simulink model "npc_controller"  (R2022a)
settings: Solver=FixedStepDiscrete  StartTime=0.0  StopTime=20  RelTol=1e-3  EnableMultiTasking=on
undefined symbols (not defined in the file): CAN_O_INT, CANA_BASE, Down, GPTRIP1SEL, GPTRIP2SEL, GPTRIP3SEL, Tsw, TZ1, TZ2, TZ3, Up
libraries: simulink x147, hdlsllib x90, c2802xlib x34, c2837xDlib x20, c280xlib x12, canmsglib x9, c2838xlib x8, idelinklib_common x3, c2806xlib x2, slpidlib x2, c28004xlib x2, c281xlib x2
(part 16 of 42)

== system npc_controller/IDLE_AND_TIMER/codegen/INITIALIZATION/clb ==
  note: // Enabling EPWM1 to enable CLB1
      | SysCtl_enablePeripheral(SYSCTL_PERIPH_CLK_EPWM1);
      | CLB_enableCLB(CLB1_BASE);
      | initTILE0(CLB1_BASE);
      |
      | // Select Global input instead of local input for all CLB IN
      | CLB_configLocalInputMux(CLB1_BASE, CLB_IN0, CLB_LOCAL_IN_MUX_GLOBAL_IN);
      | CLB_configLocalInputMux(CLB1_BASE, CLB_IN1, CLB_LOCAL_IN_MUX_GLOBAL_IN);
      | CLB_configLocalInputMux(CLB1_BASE, CLB_IN2, CLB_LOCAL_IN_MUX_GLOBAL_IN);
      | CLB_configLocalInputMux(CLB1_BASE, CLB_IN3, CLB_LOCAL_IN_MUX_GLOBAL_IN);
      | CLB_configLocalInputMux(CLB1_BASE, CLB_IN4, CLB_LOCAL_IN_MUX_GLOBAL_IN);
      | CLB_configLocalInputMux(CLB1_BASE, CLB_IN5, CLB_LOCAL_IN_MUX_GLOBAL_IN);
      | CLB_configLocalInputMux(CLB1_BASE, CLB_IN6, CLB_LOCAL_IN_MUX_GLOBAL_IN);
      | CLB_configLocalInputMux(CLB1_BASE, CLB_IN7, CLB_LOCAL_IN_MUX_GLOBAL_IN);
      |
      | // Select AUXSIG for CLBx, IN0/1/2
      | CLB_configGlobalInputMux(CLB1_BASE, CLB_IN0, CLB_GLOBAL_IN_MUX_CLB_AUXSIG0);
      | CLB_configGlobalInputMux(CLB1_BASE, CLB_IN1, CLB_GLOBAL_IN_MUX_CLB_AUXSIG1);
      | CLB_configGlobalInputMux(CLB1_BASE, CLB_IN2, CLB_GLOBAL_IN_MUX_EPWM1B);
      |
      | // Unused inputs below
      | CLB_configGlobalInputMux(CLB1_BASE, CLB_IN3, CLB_GLOBAL_IN_MUX_EPWM1A);
      | CLB_configGlobalInputMux(CLB1_BASE, CLB_IN4, CLB_GLOBAL_IN_MUX_EPWM1A);
      | CLB_configGlobalInputMux(CLB1_BASE, CLB_IN5, CLB_GLOBAL_IN_MUX_EPWM1A);
      | CLB_configGlobalInputMux(CLB1_BASE, CLB_IN6, CLB_GLOBAL_IN_MUX_EPWM1A);
      | CLB_configGlobalInputMux(CLB1_BASE, CLB_IN7, CLB_GLOBAL_IN_MUX_EPWM1A);
      |
      | // Set CLB_IN to mux external
      | CLB_configGPInputMux(CLB1_BASE, CLB_IN0, CLB_GP_IN_MUX_EXTERNAL);
      | CLB_configGPInputMux(CLB1_BASE, CLB_IN1, CLB_GP_IN_MUX_EXTERNAL);
      | CLB_configGPInputMux(CLB1_BASE, CLB_IN2, CLB_GP_IN_MUX_EXTERNAL);
      |
      | // Set unused inputs to GP register
      | CLB_configGPInputMux(CLB1_BASE, CLB_IN3, CLB_GP_IN_MUX_GP_REG);
      | CLB_configGPInputMux(CLB1_BASE, CLB_IN4, CLB_GP_IN_MUX_GP_REG);
      | CLB_configGPInputMux(CLB1_BASE, CLB_IN5, CLB_GP_IN_MUX_GP_REG);
      | CLB_configGPInputMux(CLB1_BASE, CLB_IN6, CLB_GP_IN_MUX_GP_REG);
      | CLB_configGPInputMux(CLB1_BASE, CLB_IN7, CLB_GP_IN_MUX_GP_REG);
      |
      | // Configure CLB-XBAR AUXSIG
      | XBAR_setCLBMuxConfig(XBAR_AUXSIG0, XBAR_EPWM_MUX02_CMPSS2_CTRIPH);
      | XBAR_enableCLBMux(XBAR_AUXSIG0, XBAR_MUX02);
      | XBAR_setCLBMuxConfig(XBAR_AUXSIG1, XBAR_EPWM_MUX03_CMPSS2_CTRIPL);
      | XBAR_enableCLBMux(XBAR_AUXSIG1, XBAR_MUX03);
      |
      | // Configure ePWM XBAR
      | XBAR_setEPWMMuxConfig(XBAR_TRIP4, XBAR_EPWM_MUX01_CLB1_OUT4);
      | XBAR_enableEPWMMux(XBAR_TRIP4, XBAR_MUX01);
      | XBAR_setEPWMMuxConfig(XBAR_TRIP5, XBAR_EPWM_MUX03_CLB1_OUT5);
      | XBAR_enableEPWMMux(XBAR_TRIP5, XBAR_MUX03);
  note: // Enabling EPWM1 to enable CLB1
      | SysCtl_enablePeripheral(SYSCTL_PERIPH_CLK_EPWM1);
      | CLB_enableCLB(CLB1_BASE);
      | initTILE0(CLB1_BASE);
      | CLB_enableCLB(CLB2_BASE);
      | initTILE1(CLB2_BASE);
      | CLB_enableCLB(CLB3_BASE);
      | initTILE2(CLB3_BASE);
      |
      | // Select Global input instead of local input for all CLB IN
      | CLB_configLocalInputMux(CLB1_BASE, CLB_IN0, CLB_LOCAL_IN_MUX_GLOBAL_IN);
      | CLB_configLocalInputMux(CLB1_BASE, CLB_IN1, CLB_LOCAL_IN_MUX_GLOBAL_IN);
      | CLB_configLocalInputMux(CLB1_BASE, CLB_IN2, CLB_LOCAL_IN_MUX_GLOBAL_IN);
      | CLB_configLocalInputMux(CLB1_BASE, CLB_IN3, CLB_LOCAL_IN_MUX_GLOBAL_IN);
      | CLB_configLocalInputMux(CLB1_BASE, CLB_IN4, CLB_LOCAL_IN_MUX_GLOBAL_IN);
      | CLB_configLocalInputMux(CLB1_BASE, CLB_IN5, CLB_LOCAL_IN_MUX_GLOBAL_IN);
      | CLB_configLocalInputMux(CLB1_BASE, CLB_IN6, CLB_LOCAL_IN_MUX_GLOBAL_IN);
      | CLB_configLocalInputMux(CLB1_BASE, CLB_IN7, CLB_LOCAL_IN_MUX_GLOBAL_IN);
      | CLB_configLocalInputMux(CLB2_BASE, CLB_IN0, CLB_LOCAL_IN_MUX_GLOBAL_IN);
      | CLB_configLocalInputMux(CLB2_BASE, CLB_IN1, CLB_LOCAL_IN_MUX_GLOBAL_IN);
      | CLB_configLocalInputMux(CLB2_BASE, CLB_IN2, CLB_LOCAL_IN_MUX_GLOBAL_IN);
      | CLB_configLocalInputMux(CLB2_BASE, CLB_IN3, CLB_LOCAL_IN_MUX_GLOBAL_IN);
      | CLB_configLocalInputMux(CLB2_BASE, CLB_IN4, CLB_LOCAL_IN_MUX_GLOBAL_IN);
      | CLB_configLocalInputMux(CLB2_BASE, CLB_IN5, CLB_LOCAL_IN_MUX_GLOBAL_IN);
      | CLB_configLocalInputMux(CLB2_BASE, CLB_IN6, CLB_LOCAL_IN_MUX_GLOBAL_IN);
      | CLB_configLocalInputMux(CLB2_BASE, CLB_IN7, CLB_LOCAL_IN_MUX_GLOBAL_IN);
      | CLB_configLocalInputMux(CLB3_BASE, CLB_IN0, CLB_LOCAL_IN_MUX_GLOBAL_IN);
      | CLB_configLocalInputMux(CLB3_BASE, CLB_IN1, CLB_LOCAL_IN_MUX_GLOBAL_IN);
      | CLB_configLocalInputMux(CLB3_BASE, CLB_IN2, CLB_LOCAL_IN_MUX_GLOBAL_IN);
      | CLB_configLocalInputMux(CLB3_BASE, CLB_IN3, CLB_LOCAL_IN_MUX_GLOBAL_IN);
      | CLB_configLocalInputMux(CLB3_BASE, CLB_IN4, CLB_LOCAL_IN_MUX_GLOBAL_IN);
      | CLB_configLocalInputMux(CLB3_BASE, CLB_IN5, CLB_LOCAL_IN_MUX_GLOBAL_IN);
      | CLB_configLocalInputMux(CLB3_BASE, CLB_IN6, CLB_LOCAL_IN_MUX_GLOBAL_IN);
      | CLB_configLocalInputMux(CLB3_BASE, CLB_IN7, CLB_LOCAL_IN_MUX_GLOBAL_IN);
      |
      | // Select AUXSIG for CLBx, IN0/1/2
      | CLB_configGlobalInputMux(CLB1_BASE, CLB_IN0, CLB_GLOBAL_IN_MUX_CLB_AUXSIG0);
      | CLB_configGlobalInputMux(CLB1_BASE, CLB_IN1, CLB_GLOBAL_IN_MUX_CLB_AUXSIG1);
      | CLB_configGlobalInputMux(CLB1_BASE, CLB_IN2, CLB_GLOBAL_IN_MUX_EPWM1B);
      | CLB_configGlobalInputMux(CLB2_BASE, CLB_IN0, CLB_GLOBAL_IN_MUX_CLB_AUXSIG2);
      | CLB_configGlobalInputMux(CLB2_BASE, CLB_IN1, CLB_GLOBAL_IN_MUX_CLB_AUXSIG3);
      | CLB_configGlobalInputMux(CLB2_BASE, CLB_IN2, CLB_GLOBAL_IN_MUX_EPWM3B);
      | CLB_configGlobalInputMux(CLB3_BASE, CLB_IN0, CLB_GLOBAL_IN_MUX_CLB_AUXSIG4);
      | CLB_configGlobalInputMux(CLB3_BASE, CLB_IN1, CLB_GLOBAL_IN_MUX_CLB_AUXSIG5);
      | CLB_configGlobalInputMux(CLB3_BASE, CLB_IN2, CLB_GLOBAL_IN_MUX_EPWM4B);
      |
      | // Unused inputs below
      | CLB_configGlobalInputMux(CLB1_BASE, CLB_IN3, CLB_GLOBAL_IN_MUX_EPWM1A);
      | CLB_configGlobalInputMux(CLB1_BASE, CLB_IN4, CLB_GLOBAL_IN_MUX_EPWM1A);
      | CLB_configGlobalInputMux(CLB1_BASE, CLB_IN5, CLB_GLOBAL_IN_MUX_EPWM1A);
      | CLB_configGlobalInputMux(CLB1_BASE, CLB_IN6, CLB_GLOBAL_IN_MUX_EPWM1A);
      | CLB_configGlobalInputMux(CLB1_BASE, CLB_IN7, CLB_GLOBAL_IN_MUX_EPWM1A);
      | CLB_configGlobalInputMux(CLB2_BASE, CLB_IN3, CLB_GLOBAL_IN_MUX_EPWM1A);
      | CLB_configGlobalInputMux(CLB2_BASE, CLB_IN4, CLB_GLOBAL_IN_MUX_EPWM1A);
      | CLB_configGlobalInputMux(CLB2_BASE, CLB_IN5, CLB_GLOBAL_IN_MUX_EPWM1A);
      | CLB_configGlobalInputMux(CLB2_BASE, CLB_IN6, CLB_GLOBAL_IN_MUX_EPWM1A);
      | CLB_configGlobalInputMux(CLB2_BASE, CLB_IN7, CLB_GLOBAL_IN_MUX_EPWM1A);
      | CLB_configGlobalInputMux(CLB3_BASE, CLB_IN3, CLB_GLOBAL_IN_MUX_EPWM1A);
      | CLB_configGlobalInputMux(CLB3_BASE, CLB_IN4, CLB_GLOBAL_IN_MUX_EPWM1A);
      | CLB_configGlobalInputMux(CLB3_BASE, CLB_IN5, CLB_GLOBAL_IN_MUX_EPWM1A);
      | CLB_configGlobalInputMux(CLB3_BASE, CLB_IN6, CLB_GLOBAL_IN_MUX_EPWM1A);
      | CLB_configGlobalInputMux(CLB3_BASE, CLB_IN7, CLB_GLOBAL_IN_MUX_EPWM1A);
      |
      | // Set CLB_IN to mux external
      | CLB_configGPInputMux(CLB1_BASE, CLB_IN0, CLB_GP_IN_MUX_EXTERNAL);
      | CLB_configGPInputMux(CLB1_BASE, CLB_IN1, CLB_GP_IN_MUX_EXTERNAL);
      | CLB_configGPInputMux(CLB1_BASE, CLB_IN2, CLB_GP_IN_MUX_EXTERNAL);
      | CLB_configGPInputMux(CLB2_BASE, CLB_IN0, CLB_GP_IN_MUX_EXTERNAL);
      | CLB_configGPInputMux(CLB2_BASE, CLB_IN1, CLB_GP_IN_MUX_EXTERNAL);
      | CLB_configGPInputMux(CLB2_BASE, CLB_IN2, CLB_GP_IN_MUX_EXTERNAL);
      | CLB_configGPInputMux(CLB3_BASE, CLB_IN0, CLB_GP_IN_MUX_EXTERNAL);
      | CLB_configGPInputMux(CLB3_BASE, CLB_IN1, CLB_GP_IN_MUX_EXTERNAL);
      | CLB_configGPInputMux(CLB3_BASE, CLB_IN2, CLB_GP_IN_MUX_EXTERNAL);
      |
      | // Set unused inputs to GP register
      | CLB_configGPInputMux(CLB1_BASE, CLB_IN3, CLB_GP_IN_MUX_GP_REG);
      | CLB_configGPInputMux(CLB1_BASE, CLB_IN4, CLB_GP_IN_MUX_GP_REG);
      | CLB_configGPInputMux(CLB1_BASE, CLB_IN5, CLB_GP_IN_MUX_GP_REG);
      | CLB_configGPInputMux(CLB1_BASE, CLB_IN6, CLB_GP_IN_MUX_GP_REG);
      | CLB_configGPInputMux(CLB1_BASE, CLB_IN7, CLB_GP_IN_MUX_GP_REG);
      | CLB_configGPInputMux(CLB2_BASE, CLB_IN3, CLB_GP_IN_MUX_GP_REG);
      | CLB_configGPInputMux(CLB2_BASE, CLB_IN4, CLB_GP_IN_MUX_GP_REG);
      | CLB_configGPInputMux(CLB2_BASE, CLB_IN5, CLB_GP_IN_MUX_GP_REG);
      | CLB_configGPInputMux(CLB2_BASE, CLB_IN6, CLB_GP_IN_MUX_GP_REG);
      | CLB_configGPInputMux(CLB2_BASE, CLB_IN7, CLB_GP_IN_MUX_GP_REG);
      | CLB_configGPInputMux(CLB3_BASE, CLB_IN3, CLB_GP_IN_MUX_GP_REG);
      | CLB_configGPInputMux(CLB3_BASE, CLB_IN4, CLB_GP_IN_MUX_GP_REG);
      | CLB_configGPInputMux(CLB3_BASE, CLB_IN5, CLB_GP_IN_MUX_GP_REG);
      | CLB_configGPInputMux(CLB3_BASE, CLB_IN6, CLB_GP_IN_MUX_GP_REG);
      | CLB_configGPInputMux(CLB3_BASE, CLB_IN7, CLB_GP_IN_MUX_GP_REG);
      |
      | // Configure CLB-XBAR AUXSIG
      | XBAR_setCLBMuxConfig(XBAR_AUXSIG0, XBAR_EPWM_MUX02_CMPSS2_CTRIPH);
      | XBAR_enableCLBMux(XBAR_AUXSIG0, XBAR_MUX02);
      | XBAR_setCLBMuxConfig(XBAR_AUXSIG1, XBAR_EPWM_MUX03_CMPSS2_CTRIPL);
      | XBAR_enableCLBMux(XBAR_AUXSIG1, XBAR_MUX03);
      | XBAR_setCLBMuxConfig(XBAR_AUXSIG2, XBAR_EPWM_MUX06_CMPSS4_CTRIPH);
      | XBAR_enableCLBMux(XBAR_AUXSIG2, XBAR_MUX06);
      | XBAR_setCLBMuxConfig(XBAR_AUXSIG3, XBAR_EPWM_MUX07_CMPSS4_CTRIPL);
      | XBAR_enableCLBMux(XBAR_AUXSIG3, XBAR_MUX07);
      | XBAR_setCLBMuxConfig(XBAR_AUXSIG4, XBAR_EPWM_MUX00_CMPSS1_CTRIPH);
      | XBAR_enableCLBMux(XBAR_AUXSIG4, XBAR_MUX00);
      | XBAR_setCLBMuxConfig(XBAR_AUXSIG5, XBAR_EPWM_MUX01_CMPSS1_CTRIPL);
      | XBAR_enableCLBMux(XBAR_AUXSIG5, XBAR_MUX01);
      |
      | // Configure ePWM XBAR
      | XBAR_setEPWMMuxConfig(XBAR_TRIP4, XBAR_EPWM_MUX01_CLB1_OUT4);
      | XBAR_enableEPWMMux(XBAR_TRIP4, XBAR_MUX01);
      | XBAR_setEPWMMuxConfig(XBAR_TRIP5, XBAR_EPWM_MUX03_CLB1_OUT5);
      | XBAR_enableEPWMMux(XBAR_TRIP5, XBAR_MUX03);
      | XBAR_setEPWMMuxConfig(XBAR_TRIP7, XBAR_EPWM_MUX05_CLB2_OUT4);
      | XBAR_enableEPWMMux(XBAR_TRIP7, XBAR_MUX05);
      | XBAR_setEPWMMuxConfig(XBAR_TRIP8, XBAR_EPWM_MUX07_CLB2_OUT5);
      | XBAR_enableEPWMMux(XBAR_TRIP8, XBAR_MUX07);
      | XBAR_setEPWMMuxConfig(XBAR_TRIP9, XBAR_EPWM_MUX09_CLB3_OUT4);
      | XBAR_enableEPWMMux(XBAR_TRIP9, XBAR_MUX09);
      | XBAR_setEPWMMuxConfig(XBAR_TRIP10, XBAR_EPWM_MUX11_CLB3_OUT5);
      | XBAR_enableEPWMMux(XBAR_TRIP10, XBAR_MUX11);
  note: // Enabling EPWM1 to enable CLB1
      | SysCtl_enablePeripheral(SYSCTL_PERIPH_CLK_EPWM1);
      | CLB_enableCLB(CLB1_BASE);
      | initTILE0(CLB1_BASE);
      | CLB_enableCLB(CLB2_BASE);
      | initTILE1(CLB2_BASE);
      | CLB_enableCLB(CLB3_BASE);
      | initTILE2(CLB3_BASE);
      |
      | // Select Global input instead of local input for all CLB IN
      | CLB_configLocalInputMux(CLB1_BASE, CLB_IN0, CLB_LOCAL_IN_MUX_GLOBAL_IN);
      | CLB_configLocalInputMux(CLB1_BASE, CLB_IN1, CLB_LOCAL_IN_MUX_GLOBAL_IN);
      | CLB_configLocalInputMux(CLB1_BASE, CLB_IN2, CLB_LOCAL_IN_MUX_GLOBAL_IN);
      | CLB_configLocalInputMux(CLB1_BASE, CLB_IN3, CLB_LOCAL_IN_MUX_GLOBAL_IN);
      | CLB_configLocalInputMux(CLB1_BASE, CLB_IN4, CLB_LOCAL_IN_MUX_GLOBAL_IN);
      | CLB_configLocalInputMux(CLB1_BASE, CLB_IN5, CLB_LOCAL_IN_MUX_GLOBAL_IN);
      | CLB_configLocalInputMux(CLB1_BASE, CLB_IN6, CLB_LOCAL_IN_MUX_GLOBAL_IN);
      | CLB_configLocalInputMux(CLB1_BASE, CLB_IN7, CLB_LOCAL_IN_MUX_GLOBAL_IN);
      | CLB_configLocalInputMux(CLB2_BASE, CLB_IN0, CLB_LOCAL_IN_MUX_GLOBAL_IN);
      | CLB_configLocalInputMux(CLB2_BASE, CLB_IN1, CLB_LOCAL_IN_MUX_GLOBAL_IN);
      | CLB_configLocalInputMux(CLB2_BASE, CLB_IN2, CLB_LOCAL_IN_MUX_GLOBAL_IN);
      | CLB_configLocalInputMux(CLB2_BASE, CLB_IN3, CLB_LOCAL_IN_MUX_GLOBAL_IN);
      | CLB_configLocalInputMux(CLB2_BASE, CLB_IN4, CLB_LOCAL_IN_MUX_GLOBAL_IN);
      | CLB_configLocalInputMux(CLB2_BASE, CLB_IN5, CLB_LOCAL_IN_MUX_GLOBAL_IN);
      | CLB_configLocalInputMux(CLB2_BASE, CLB_IN6, CLB_LOCAL_IN_MUX_GLOBAL_IN);
      | CLB_configLocalInputMux(CLB2_BASE, CLB_IN7, CLB_LOCAL_IN_MUX_GLOBAL_IN);
      | CLB_configLocalInputMux(CLB3_BASE, CLB_IN0, CLB_LOCAL_IN_MUX_GLOBAL_IN);
      | CLB_configLocalInputMux(CLB3_BASE, CLB_IN1, CLB_LOCAL_IN_MUX_GLOBAL_IN);
      | CLB_configLocalInputMux(CLB3_BASE, CLB_IN2, CLB_LOCAL_IN_MUX_GLOBAL_IN);
      | CLB_configLocalInputMux(CLB3_BASE, CLB_IN3, CLB_LOCAL_IN_MUX_GLOBAL_IN);
      | CLB_configLocalInputMux(CLB3_BASE, CLB_IN4, CLB_LOCAL_IN_MUX_GLOBAL_IN);
      | CLB_configLocalInputMux(CLB3_BASE, CLB_IN5, CLB_LOCAL_IN_MUX_GLOBAL_IN);
      | CLB_configLocalInputMux(CLB3_BASE, CLB_IN6, CLB_LOCAL_IN_MUX_GLOBAL_IN);
      | CLB_configLocalInputMux(CLB3_BASE, CLB_IN7, CLB_LOCAL_IN_MUX_GLOBAL_IN);
      |
      | // Select AUXSIG for CLBx, IN0/1/2
      | CLB_configGlobalInputMux(CLB1_BASE, CLB_IN0, CLB_GLOBAL_IN_MUX_CLB_AUXSIG0);
      | CLB_configGlobalInputMux(CLB1_BASE, CLB_IN1, CLB_GLOBAL_IN_MUX_CLB_AUXSIG1);
      | CLB_configGlobalInputMux(CLB1_BASE, CLB_IN2, CLB_GLOBAL_IN_MUX_EPWM1B);
      |
      | CLB_configGlobalInputMux(CLB2_BASE, CLB_IN0, CLB_GLOBAL_IN_MUX_CLB_AUXSIG2);
      | CLB_configGlobalInputMux(CLB2_BASE, CLB_IN1, CLB_GLOBAL_IN_MUX_CLB_AUXSIG3);
      | CLB_configGlobalInputMux(CLB2_BASE, CLB_IN2, CLB_GLOBAL_IN_MUX_EPWM3B);
      |
      | CLB_configGlobalInputMux(CLB3_BASE, CLB_IN0, CLB_GLOBAL_IN_MUX_CLB_AUXSIG4);
      | CLB_configGlobalInputMux(CLB3_BASE, CLB_IN1, CLB_GLOBAL_IN_MUX_CLB_AUXSIG5);
      | CLB_configGlobalInputMux(CLB3_BASE, CLB_IN2, CLB_GLOBAL_IN_MUX_EPWM4B);
      |
      | // Unused inputs below
      | CLB_configGlobalInputMux(CLB1_BASE, CLB_IN3, CLB_GLOBAL_IN_MUX_EPWM1A);
      | CLB_configGlobalInputMux(CLB1_BASE, CLB_IN4, CLB_GLOBAL_IN_MUX_EPWM1A);
      | CLB_configGlobalInputMux(CLB1_BASE, CLB_IN5, CLB_GLOBAL_IN_MUX_EPWM1A);
      | CLB_configGlobalInputMux(CLB1_BASE, CLB_IN6, CLB_GLOBAL_IN_MUX_EPWM1A);
      | CLB_configGlobalInputMux(CLB1_BASE, CLB_IN7, CLB_GLOBAL_IN_MUX_EPWM1A);
      | CLB_configGlobalInputMux(CLB2_BASE, CLB_IN3, CLB_GLOBAL_IN_MUX_EPWM1A);
      | CLB_configGlobalInputMux(CLB2_BASE, CLB_IN4, CLB_GLOBAL_IN_MUX_EPWM1A);
      | CLB_configGlobalInputMux(CLB2_BASE, CLB_IN5, CLB_GLOBAL_IN_MUX_EPWM1A);
      | CLB_configGlobalInputMux(CLB2_BASE, CLB_IN6, CLB_GLOBAL_IN_MUX_EPWM1A);
      | CLB_configGlobalInputMux(CLB2_BASE, CLB_IN7, CLB_GLOBAL_IN_MUX_EPWM1A);
      | CLB_configGlobalInputMux(CLB3_BASE, CLB_IN3, CLB_GLOBAL_IN_MUX_EPWM1A);
      | CLB_configGlobalInputMux(CLB3_BASE, CLB_IN4, CLB_GLOBAL_IN_MUX_EPWM1A);
      | CLB_configGlobalInputMux(CLB3_BASE, CLB_IN5, CLB_GLOBAL_IN_MUX_EPWM1A);
      | CLB_configGlobalInputMux(CLB3_BASE, CLB_IN6, CLB_GLOBAL_IN_MUX_EPWM1A);
      | CLB_configGlobalInputMux(CLB3_BASE, CLB_IN7, CLB_GLOBAL_IN_MUX_EPWM1A);
      |
      | // Set CLB_IN to mux external
      | CLB_configGPInputMux(CLB1_BASE, CLB_IN0, CLB_GP_IN_MUX_EXTERNAL);
      | CLB_configGPInputMux(CLB1_BASE, CLB_IN1, CLB_GP_IN_MUX_EXTERNAL);
      | CLB_configGPInputMux(CLB1_BASE, CLB_IN2, CLB_GP_IN_MUX_EXTERNAL);
      | CLB_configGPInputMux(CLB2_BASE, CLB_IN0, CLB_GP_IN_MUX_EXTERNAL);
      | CLB_configGPInputMux(CLB2_BASE, CLB_IN1, CLB_GP_IN_MUX_EXTERNAL);
      | CLB_configGPInputMux(CLB2_BASE, CLB_IN2, CLB_GP_IN_MUX_EXTERNAL);
      | CLB_configGPInputMux(CLB3_BASE, CLB_IN0, CLB_GP_IN_MUX_EXTERNAL);
      | CLB_configGPInputMux(CLB3_BASE, CLB_IN1, CLB_GP_IN_MUX_EXTERNAL);
      | CLB_configGPInputMux(CLB3_BASE, CLB_IN2, CLB_GP_IN_MUX_EXTERNAL);
      |
      | // Set unused inputs to GP register
      | CLB_configGPInputMux(CLB1_BASE, CLB_IN3, CLB_GP_IN_MUX_GP_REG);
      | CLB_configGPInputMux(CLB1_BASE, CLB_IN4, CLB_GP_IN_MUX_GP_REG);
      | CLB_configGPInputMux(CLB1_BASE, CLB_IN5, CLB_GP_IN_MUX_GP_REG);
      | CLB_configGPInputMux(CLB1_BASE, CLB_IN6, CLB_GP_IN_MUX_GP_REG);
      | CLB_configGPInputMux(CLB1_BASE, CLB_IN7, CLB_GP_IN_MUX_GP_REG);
      | CLB_configGPInputMux(CLB2_BASE, CLB_IN3, CLB_GP_IN_MUX_GP_REG);
      | CLB_configGPInputMux(CLB2_BASE, CLB_IN4, CLB_GP_IN_MUX_GP_REG);
      | CLB_configGPInputMux(CLB2_BASE, CLB_IN5, CLB_GP_IN_MUX_GP_REG);
      | CLB_configGPInputMux(CLB2_BASE, CLB_IN6, CLB_GP_IN_MUX_GP_REG);
      | CLB_configGPInputMux(CLB2_BASE, CLB_IN7, CLB_GP_IN_MUX_GP_REG);
      | CLB_configGPInputMux(CLB3_BASE, CLB_IN3, CLB_GP_IN_MUX_GP_REG);
      | CLB_configGPInputMux(CLB3_BASE, CLB_IN4, CLB_GP_IN_MUX_GP_REG);
      | CLB_configGPInputMux(CLB3_BASE, CLB_IN5, CLB_GP_IN_MUX_GP_REG);
      | CLB_configGPInputMux(CLB3_BASE, CLB_IN6, CLB_GP_IN_MUX_GP_REG);
      | CLB_configGPInputMux(CLB3_BASE, CLB_IN7, CLB_GP_IN_MUX_GP_REG);
      |
      | // Configure CLB-XBAR AUXSIG
      | XBAR_setCLBMuxConfig(XBAR_AUXSIG0,XBAR_EPWM_MUX00_CMPSS1_CTRIPH);
      | XBAR_enableCLBMux(XBAR_AUXSIG0, XBAR_MUX00);
      | XBAR_setCLBMuxConfig(XBAR_AUXSIG1, XBAR_EPWM_MUX01_CMPSS1_CTRIPL);
      | XBAR_enableCLBMux(XBAR_AUXSIG1, XBAR_MUX01);
      |
      |
      | XBAR_setCLBMuxConfig(XBAR_AUXSIG2, XBAR_EPWM_MUX06_CMPSS4_CTRIPH);
      | XBAR_enableCLBMux(XBAR_AUXSIG2, XBAR_MUX06);
      | XBAR_setCLBMuxConfig(XBAR_AUXSIG3, XBAR_EPWM_MUX07_CMPSS4_CTRIPL);
      | XBAR_enableCLBMux(XBAR_AUXSIG3, XBAR_MUX07);
      |
      |
      | XBAR_setCLBMuxConfig(XBAR_AUXSIG4, XBAR_EPWM_MUX02_CMPSS2_CTRIPH );
      | XBAR_enableCLBMux(XBAR_AUXSIG4, XBAR_MUX02);
      | XBAR_setCLBMuxConfig(XBAR_AUXSIG5, XBAR_EPWM_MUX03_CMPSS2_CTRIPL);
      | XBAR_enableCLBMux(XBAR_AUXSIG5, XBAR_MUX03);
      |
      | // Configure ePWM XBAR
      | XBAR_setEPWMMuxConfig(XBAR_TRIP4, XBAR_EPWM_MUX01_CLB1_OUT4);
      | XBAR_enableEPWMMux(XBAR_TRIP4, XBAR_MUX01);
      | XBAR_setEPWMMuxConfig(XBAR_TRIP5, XBAR_EPWM_MUX03_CLB1_OUT5);
      | XBAR_enableEPWMMux(XBAR_TRIP5, XBAR_MUX03);
      | XBAR_setEPWMMuxConfig(XBAR_TRIP7, XBAR_EPWM_MUX05_CLB2_OUT4);
      | XBAR_enableEPWMMux(XBAR_TRIP7, XBAR_MUX05);
      | XBAR_setEPWMMuxConfig(XBAR_TRIP8, XBAR_EPWM_MUX07_CLB2_OUT5);
      | XBAR_enableEPWMMux(XBAR_TRIP8, XBAR_MUX07);
      | XBAR_setEPWMMuxConfig(XBAR_TRIP9, XBAR_EPWM_MUX09_CLB3_OUT4);
      | XBAR_enableEPWMMux(XBAR_TRIP9, XBAR_MUX09);
      | XBAR_setEPWMMuxConfig(XBAR_TRIP10, XBAR_EPWM_MUX11_CLB3_OUT5);
      | XBAR_enableEPWMMux(XBAR_TRIP10, XBAR_MUX11);
  function : TriggerPort  TriggerType=function-call  VariantControl=Variant
  System Initialize1 : Subsystem  Commented=on  mask(System Initialize){ShowInLibBrowser=0}
      mask prompts: ShowInLibBrowser "Simulink:masks:CustCodeMaskParam1_MP"
      settings: CopyFcn=cccopyfcn(gcb)  OpenFcn=ccopenfcn('System Initialize Function')
      mask Help: eval('feval(''rtwprivate'',''rtwhelpview'',''rtw_sys_initialize_block'')');
      mask Display: disp('System\nInitialize');
  System Initialize2 : Subsystem  mask(System Initialize){ShowInLibBrowser=0}
      mask prompts: ShowInLibBrowser "Simulink:masks:CustCodeMaskParam1_MP"
      settings: CopyFcn=cccopyfcn(gcb)  OpenFcn=ccopenfcn('System Initialize Function')
      mask Help: eval('feval(''rtwprivate'',''rtwhelpview'',''rtw_sys_initialize_block'')');
      mask Display: disp('System\nInitialize');
  System Initialize8 : Subsystem  Commented=on  mask(System Initialize){ShowInLibBrowser=0}
      mask prompts: ShowInLibBrowser "Simulink:masks:CustCodeMaskParam1_MP"
      settings: CopyFcn=cccopyfcn(gcb)  OpenFcn=ccopenfcn('System Initialize Function')
      mask Help: eval('feval(''rtwprivate'',''rtwhelpview'',''rtw_sys_initialize_block'')');
      mask Display: disp('System\nInitialize');

== system npc_controller/IDLE_AND_TIMER/codegen/INITIALIZATION/cmpss ==
  note: Note: After swapping
      | ADCINA4/CMPIN2P ICSA_AD
      | ADCIN14/CMPIN4P ICSB_AD
      | ADCINA2/CMPIN1P ICSC_AD
  function : TriggerPort  TriggerType=function-call  VariantControl=Variant
  10A inst2 : Constant  Commented=on  Value=1.65+0.2+0.02
  20A inst1 : Constant  Commented=on  Value=1.65+0.4+0.05
  25A inst4 : Constant  Value=1.65+0.5+0.05
  2A inst3 : Constant  Commented=on  Value=1.65+0.04+0.02
  30A inst1 : Constant  Value=1.65+0.6+0.05
  30A inst2 : Constant  Value=1.65+0.6+0.05
  30A inst3 : Constant  Value=1.65+0.6+0.05
  3A inst4 : Constant  Commented=on  Value=1.65+0.06+0.02
  5A inst1 : Constant  Commented=on  Value=1.65+0.09+0.05
  5A inst4 : Constant  Commented=on  Value=1.65+0.1+0.02
  CMPSS1H : c2837xDlib/CMPSS  Module=CMPSS1_COMPH  NegativeInput=Internal DAC  DacValueSourceSel=DAC module  DacValueVia=Input port  DACHValue=2234  DACLValue=0  RampMaxRefVal=0  RampDecVal=0  RampDelayVal=0  EnableLatchOut=off  EnableLatchClear=off  SampleTime=-1
      settings: SourceProductBaseCode=TIC2000
  CMPSS1L : c2837xDlib/CMPSS  Module=CMPSS1_COMPL  NegativeInput=Internal DAC  DacValueSourceSel=DAC module  DacValueVia=Input port  DACHValue=2234  DACLValue=0  RampMaxRefVal=0  RampDecVal=0  RampDelayVal=0  EnableLatchOut=off  EnableLatchClear=off  SampleTime=-1
      settings: SourceProductBaseCode=TIC2000
  CMPSS2H : c2837xDlib/CMPSS  Module=CMPSS2_COMPH  NegativeInput=Internal DAC  DacValueSourceSel=DAC module  DacValueVia=Input port  DACHValue=2234  DACLValue=0  RampMaxRefVal=0  RampDecVal=0  RampDelayVal=0  EnableLatchOut=off  EnableLatchClear=off  SampleTime=-1
      settings: SourceProductBaseCode=TIC2000
  CMPSS2L : c2837xDlib/CMPSS  Module=CMPSS2_COMPL  NegativeInput=Internal DAC  DacValueSourceSel=DAC module  DacValueVia=Input port  DACHValue=2234  DACLValue=0  RampMaxRefVal=0  RampDecVal=0  RampDelayVal=0  EnableLatchOut=off  EnableLatchClear=off  SampleTime=-1
      settings: SourceProductBaseCode=TIC2000
  CMPSS4H : c2837xDlib/CMPSS  Module=CMPSS4_COMPH  NegativeInput=Internal DAC  DacValueSourceSel=DAC module  DacValueVia=Input port  DACHValue=2234  DACLValue=0  RampMaxRefVal=0  RampDecVal=0  RampDelayVal=0  EnableLatchOut=off  EnableLatchClear=off  SampleTime=-1
      settings: SourceProductBaseCode=TIC2000
  CMPSS4L : c2837xDlib/CMPSS  Module=CMPSS4_COMPL  NegativeInput=Internal DAC  DacValueSourceSel=DAC module  DacValueVia=Input port  DACHValue=2234  DACLValue=0  RampMaxRefVal=0  RampDecVal=0  RampDelayVal=0  EnableLatchOut=off  EnableLatchClear=off  SampleTime=-1
      settings: SourceProductBaseCode=TIC2000
  Constant1 : Constant  Commented=on  Value=1.65-0.2+0.02
  Constant2 : Constant  Commented=on  Value=1.65-0.09+0.05
  Constant3 : Constant  Value=1.65-0.6+0.05
  Constant4 : Constant  Commented=on  Value=1.65-0.04+0.02
  Constant5 : Constant  Commented=on  Value=1.65-0.1+0.02
  Constant6 : Constant  Value=1.65-0.6+0.05
  Constant7 : Constant  Value=1.65-0.6+0.05
  Constant8 : Constant  Value=1.65-0.5+0.05
  Constant9 : Constant  Commented=on  Value=1.65-0.06+0.02
  Gain{1..6} (6 alike) : Gain  Gain=1240.91
  Gain7 : Gain  Commented=on  Gain=1240.91
  Gain8 : Gain  Commented=on  Gain=1240.91
  wires:
  Gain2/1 -> CMPSS4H/1
  Gain3/1 -> CMPSS4L/1
  30A inst1/1 -> Gain2/1
  Constant6/1 -> Gain3/1
  Gain4/1 -> CMPSS1H/1
  Gain5/1 -> CMPSS1L/1
  Gain1/1 -> CMPSS2H/1
  Gain6/1 -> CMPSS2L/1
  Constant3/1 -> Gain6/1
  30A inst2/1 -> Gain1/1
  2A inst3/1 -> Gain7/1
  Constant4/1 -> Gain8/1
  Constant7/1 -> Gain5/1
  30A inst3/1 -> Gain4/1

== system npc_controller/IDLE_AND_TIMER/codegen/INITIALIZATION/epwm ==
  note: Note:
      |
      | Function PWM # GPIO # LAUNCHPAD PIN #
      |
      | Synci EPWM1A GPIO0 J4.40
      | EPWM1B GPIO1 J4.39
      |
      | TZ GPIO62 XX
      |
      | a_s1 EPWM6B GPIO11 J8.75
      | a_s2 EPWM7B GPIO13 XX
      | a_s3 EPWM6A GPIO10 J8.76
      | a_s4 EPWM7A GPIO12 XX
      |
      | b_s1 EPWM8B GPIO15 J8.73
      | b_s2 EPWM9B GPIO17 XX
      | b_s3 EPWM8A GPIO14 J8.74
      | b_s4 EPWM9A GPIO16 J4.33
      |
      | c_s1 EPWM10B GPIO19 J1.3
      | c_s2 EPWM11B GPIO21 XX
      | c_s3 EPWM10A GPIO18 J1.4
      | c_s4 EPWM11A GPIO20 XX
  note: /*Initialize pwm sync*/
      | EALLOW;
      | XBAR_setInputPin(XBAR_INPUT5, 0); //EXTSYNC1 from PWM1A
      | SyncSocRegs.SYNCSELECT.bit.EPWM4SYNCIN = 0b101; //Sync PWM4 group to EXTSYNC1
      | SyncSocRegs.SYNCSELECT.bit.EPWM7SYNCIN = 0b101; //Sync PWM7 group to EXTSYNC1
      | SyncSocRegs.SYNCSELECT.bit.EPWM10SYNCIN = 0b101; //Sync PWM10 group to EXTSYNC1
      | EDIS;
      |
      | /*Force PWM to LOW*/
      | EPwm2Regs.AQCSFRC.bit.CSFA = (uint16_T)(0b01);
      | EPwm2Regs.AQCSFRC.bit.CSFB = (uint16_T)(0b01);
      | EPwm7Regs.AQCSFRC.bit.CSFA = (uint16_T)(0b01);
      | EPwm7Regs.AQCSFRC.bit.CSFB = (uint16_T)(0b01);
      | EPwm8Regs.AQCSFRC.bit.CSFA = (uint16_T)(0b01);
      | EPwm8Regs.AQCSFRC.bit.CSFB = (uint16_T)(0b01);
      | EPwm9Regs.AQCSFRC.bit.CSFA = (uint16_T)(0b01);
      | EPwm9Regs.AQCSFRC.bit.CSFB = (uint16_T)(0b01);
      | EPwm10Regs.AQCSFRC.bit.CSFA = (uint16_T)(0b01);
      | EPwm10Regs.AQCSFRC.bit.CSFB = (uint16_T)(0b01);
      | EPwm11Regs.AQCSFRC.bit.CSFA = (uint16_T)(0b01);
      | EPwm11Regs.AQCSFRC.bit.CSFB = (uint16_T)(0b01);
  note: Note:
      | PWM grouping:
      | Group 1: 1, 2, 3 (only sync option is EXTSYNC1, no need to configure)
      | Group 4: 4, 5, 6
      | Group 7: 7, 8
      |
      | All will sync to EPWM1
  note: Note:
      | TZCCTL
      | 0b00 - High impedance
      | 0b01 - Force to HIGH
      | 0b10 - Force to LOW
      | 0b11 - Do nothing
      |
      | AQCSFRC
      | 0b00 - disables forced PWM
      | 0b01 - forces PWM to LOW
      | 0b10 - forces PWM to  HIGH
  function : TriggerPort  TriggerType=function-call  VariantControl=Variant
  System Initialize3 : Subsystem  mask(System Initialize){ShowInLibBrowser=0}
      mask prompts: ShowInLibBrowser "Simulink:masks:CustCodeMaskParam1_MP"
      settings: CopyFcn=cccopyfcn(gcb)  OpenFcn=ccopenfcn('System Initialize Function')
      mask Help: eval('feval(''rtwprivate'',''rtwhelpview'',''rtw_sys_initialize_block'')');
      mask Display: disp('System\nInitialize');

== system npc_controller/IDLE_AND_TIMER/codegen/INITIALIZATION/epwm1 ==
  note: /*Initialize pwm sync*/
      | EALLOW;
      | XBAR_setInputPin(XBAR_INPUT5, 0); //EXTSYNC1 from PWM1A
      | SyncSocRegs.SYNCSELECT.bit.EPWM4SYNCIN = 0b101; //Sync PWM4 group to EXTSYNC1
      | SyncSocRegs.SYNCSELECT.bit.EPWM7SYNCIN = 0b101; //Sync PWM7 group to EXTSYNC1
      | SyncSocRegs.SYNCSELECT.bit.EPWM10SYNCIN = 0b101; //Sync PWM10 group to EXTSYNC1
      | EDIS;
      |
      | /*Force PWM to LOW*/
      | //EPwm6Regs.AQCSFRC.bit.CSFA = (uint16_T)(0b01);
      | //EPwm6Regs.AQCSFRC.bit.CSFB = (uint16_T)(0b01);
      | //EPwm7Regs.AQCSFRC.bit.CSFA = (uint16_T)(0b01);
      | //EPwm7Regs.AQCSFRC.bit.CSFB = (uint16_T)(0b01);
      | //EPwm8Regs.AQCSFRC.bit.CSFA = (uint16_T)(0b01);
      | //EPwm8Regs.AQCSFRC.bit.CSFB = (uint16_T)(0b01);
      | //EPwm9Regs.AQCSFRC.bit.CSFA = (uint16_T)(0b01);
      | //EPwm9Regs.AQCSFRC.bit.CSFB = (uint16_T)(0b01);
      | //EPwm10Regs.AQCSFRC.bit.CSFA = (uint16_T)(0b01);
      | //EPwm10Regs.AQCSFRC.bit.CSFB = (uint16_T)(0b01);
      | //EPwm11Regs.AQCSFRC.bit.CSFA = (uint16_T)(0b01);
      | //EPwm11Regs.AQCSFRC.bit.CSFB = (uint16_T)(0b01);
  note: Note:
      | AQCSFRC
      | 0b00 - disables forced PWM
      | 0b01 - forces PWM to LOW
      | 0b10 - forces PWM to  HIGH
  note: Note:
      | PWM grouping:
      | Group 1: 1, 2, 3 (only sync option is EXTSYNC1, no need to configure)
      | Group 4: 4, 5, 6
      | Group 7: 7, 8
      |
      | All will sync to EPWM1
  note: /*Initialize pwm sync*/
      | EALLOW;
      | XBAR_setInputPin(XBAR_INPUT5, 0); //EXTSYNC1 from PWM1A
      | SyncSocRegs.SYNCSELECT.bit.EPWM4SYNCIN = 0b101; //Sync PWM4 group to EXTSYNC1
      | SyncSocRegs.SYNCSELECT.bit.EPWM7SYNCIN = 0b101; //Sync PWM7 group to EXTSYNC1
      | SyncSocRegs.SYNCSELECT.bit.EPWM10SYNCIN = 0b101; //Sync PWM10 group to EXTSYNC1
      | EDIS;
      |
      | /*Force PWM to LOW*/
      | EPwm6Regs.AQCSFRC.bit.CSFA = (uint16_T)(0b01);
      | EPwm6Regs.AQCSFRC.bit.CSFB = (uint16_T)(0b01);
      | EPwm7Regs.AQCSFRC.bit.CSFA = (uint16_T)(0b01);
      | EPwm7Regs.AQCSFRC.bit.CSFB = (uint16_T)(0b01);
      | EPwm8Regs.AQCSFRC.bit.CSFA = (uint16_T)(0b01);
      | EPwm8Regs.AQCSFRC.bit.CSFB = (uint16_T)(0b01);
      | EPwm9Regs.AQCSFRC.bit.CSFA = (uint16_T)(0b01);
      | EPwm9Regs.AQCSFRC.bit.CSFB = (uint16_T)(0b01);
      | EPwm10Regs.AQCSFRC.bit.CSFA = (uint16_T)(0b01);
      | EPwm10Regs.AQCSFRC.bit.CSFB = (uint16_T)(0b01);
      | EPwm11Regs.AQCSFRC.bit.CSFA = (uint16_T)(0b01);
      | EPwm11Regs.AQCSFRC.bit.CSFB = (uint16_T)(0b01);
  note: Note:
      |
      | Function PWM # GPIO # LAUNCHPAD PIN #
      |
      | Synci EPWM1A GPIO0 J4.40
      | EPWM1B GPIO1 J4.39
      |
      | TZ GPIO62 XX
      |
      | a_s1 EPWM6B GPIO11 J8.75
      | a_s2 EPWM7B GPIO13 XX
      | a_s3 EPWM6A GPIO10 J8.76
      | a_s4 EPWM7A GPIO12 XX
      |
      | b_s1 EPWM8B GPIO15 J8.73
      | b_s2 EPWM9B GPIO17 XX
      | b_s3 EPWM8A GPIO14 J8.74
      | b_s4 EPWM9A GPIO16 J4.33
      |
      | c_s1 EPWM10B GPIO19 J1.3
      | c_s2 EPWM11B GPIO21 XX
      | c_s3 EPWM10A GPIO18 J1.4
      | c_s4 EPWM11A GPIO20 XX
  function : TriggerPort  TriggerType=function-call  VariantControl=Variant
  System Initialize1 : Subsystem  Commented=on  mask(System Initialize){ShowInLibBrowser=0}
      mask prompts: ShowInLibBrowser "Simulink:masks:CustCodeMaskParam1_MP"
      settings: CopyFcn=cccopyfcn(gcb)  OpenFcn=ccopenfcn('System Initialize Function')
      mask Help: eval('feval(''rtwprivate'',''rtwhelpview'',''rtw_sys_initialize_block'')');
      mask Display: disp('System\nInitialize');
  System Initialize3 : Subsystem  mask(System Initialize){ShowInLibBrowser=0}
      mask prompts: ShowInLibBrowser "Simulink:masks:CustCodeMaskParam1_MP"
      settings: CopyFcn=cccopyfcn(gcb)  OpenFcn=ccopenfcn('System Initialize Function')
      mask Help: eval('feval(''rtwprivate'',''rtwhelpview'',''rtw_sys_initialize_block'')');
      mask Display: disp('System\nInitialize');

== system npc_controller/IDLE_AND_TIMER/codegen/INITIALIZATION/orps&relay ==
  note: Note:
      | Period: 65kHz
      | Deadband: 250ns
  function : TriggerPort  TriggerType=function-call  VariantControl=Variant
  ePWM2 - ORPS1 : c2802xlib/ePWM  Commented=on  PwmType=C2000_Type4  useModule=ePWM2  ePWMxLINKTBPRD=Not Linked  periodUnits=Clock cycles  timerSource=Specify via dialog  timerPeriod_clk=1000  timerPeriod_sec=0.0001  tbshadow=Counter equals to zero  countingMode=Up-Down  phaseActiveEnable=Disable  phaseDirection=Count down after sync  phaseActive=0  synchronizationEnable=off  dcaevt1Sync=off  dcbevt1Sync=off  synchronizationOption=Counter equals to zero (CTR=Zero)  perSynchronizationOption=Counter equals to period (CTR=PRD)  clockPrescale=1  HSclockPrescale=1  enswap=off  ePWMxAStatus=on  ePWMxAactionLogic1=Do nothing  ePWMxAactionLogic2=Do nothing  ePWMxAactionLogic3=Clear  ePWMxAactionLogic4=Set  ePWMxAactionLogic5=Do nothing  ePWMxAactionLogic6=Do nothing  ePWMxACSFenable=off  ePWMxACSFvalue=Forcing disable  ePWMxASFreload=Period  ePWMxBStatus=on  ePWMxBactionLogic1=Do nothing  ePWMxBactionLogic2=Do nothing  ePWMxBactionLogic3=Do nothing  ePWMxBactionLogic4=Do nothing  ePWMxBactionLogic5=Set  ePWMxBactionLogic6=Clear  ePWMxBCSFenable=off  ePWMxBCSFvalue=Forcing disable  ePWMxBSFreload=Period  ePWNxBOutWay=off  ePWMxLINKCMPA=Not Linked  CMPAUnits=Clock cycles  CMPASource=Specify via dialog  CMPAValue_per=50  CMPAValue_clk=500-25  enCMPAshadow=Counter equals to period (CTR=PRD)  ePWMxLINKCMPB=Not Linked  CMPBUnits=Clock cycles  CMPBSource=Specify via dialog  CMPBValue_per=50  CMPBValue_clk=500+25  enCMPBshadow=Counter equals to period (CTR=PRD)  ePWMxLINKCMPC=Not Linked  CMPCUnits=Clock cycles  CMPCSource=Specify via dialog  CMPCValue_per=50  CMPCValue_clk=32000  enCMPCshadow=Counter equals to zero (CTR=Zero)  ePWMxLINKCMPD=Not Linked  CMPDUnits=Clock cycles  CMPDSource=Specify via dialog  CMPDValue_per=50  CMPDValue_clk=32000  enCMPDshadow=Counter equals to zero (CTR=Zero)  enableDBePWMxA=off  enableDBePWMxB=off  enhalfcycle=off  DBpolarity=Active high (AH)  DBedgeDelay=Positive  DBSource_ePWMxA=ePWMxA  DBSource_ePWMxB=ePWMxA  DBPeriodUnits=Clock cycles  DBperiodSource=Specify via dialog  REDperiod=0  FEDperiod=0  REDperiod_sec=0  FEDperiod_sec=0  LoadModeDBRED=Immediate without using shadow  LoadModeDBFED=Immediate without using shadow  adcstartModuleA=off  adcrequestEventA=First event  adcstartEventA=Digital Compare Module A Event 1 start of conversion (DCAEVT1.soc)  adcstartEventA_type2=Counter equals to zero (CTR=Zero)  adcstartModuleB=off  adcrequestEventB=First event  adcstartEventB=Counter equals to zero (CTR=Zero)  adcstartEventB_type2=Counter equals to zero (CTR=Zero)  intEn=off  intPrd=First event  intSel=Counter equals to zero (CTR=Zero)  intSel_type2=Counter equals to zero (CTR=Zero)  hrpe=off  enHRPWM=off  HRPWM_LoadMode=Counter equals to period (CTR=PRD)  HRPWM_CTLMode=Duty or Period control mode  HRPWM_EDGMode=Both edge  hrpeb=off  enHRPWMB=off  HRPWM_LoadModeB=Counter equals to zero (CTR=ZERO)  HRPWM_CTLModeB=Duty or Period control mode  HRPWM_EDGModeB=Both edge  enHRDBRED=off  enHRDBFED=off  enSFO=on  enautoconv=on  chopperEnable=off  chopperFrequency=1  chopperFirstwidth=1  chopperDuty=12.5%  tripZonesource=Specify via dialog  tzselOSHT1=off  tzselOSHT2=off  tzselOSHT3=off  tzselOSHDCAEV1=off  tzselOSHDCBEV1=off  tzselCBC1=off  tzselCBC2=off  tzselCBC3=off  tzselCBCDCAEV2=off  tzselCBCDCBEV2=off  tzselOSHT4=off  tzselOSHT5=off  tzselOSHT6=off  tzselCBC4=off  tzselCBC5=off  tzselCBC6=off  enTzOstIntr=off  enTzCbcIntr=off  enTzDCAEVT1Intr=off  enTzDCAEVT2Intr=off  enTzDCBEVT1Intr=off  enTzDCBEVT2Intr=off  ePWMxAforced=No action  ePWMxBforced=No action  DCAEVT1forced=No action  DCBEVT1forced=No action  DCAEVT2forced=No action  DCBEVT2forced=No action  dcah=Trip Zone 1 input (TZ1)  dcal=Trip Zone 2 input (TZ2)  dcbh=Trip Zone 1 input (TZ1)  dcbl=Trip Zone 2 input (TZ2)  dcah_type2=GPTRIP1SEL/(TZ1)  dcal_type2=GPTRIP2SEL/(TZ2)  dcbh_type2=GPTRIP1SEL/(TZ1)  dcbl_type2=GPTRIP2SEL/(TZ2)  gendcaevt1=Event disabled  gendcaevt2=Event disabled  gendcbevt1=Event disabled  gendcbevt2=Event disabled  dcaevt1src=DCAEVT1 with sync  dcaevt2src=DCAEVT2 with sync  dcbevt1src=DCBEVT1 with sync  dcbevt2src=DCBEVT2 with sync  pulsesel=Counter equals to zero (CTR=Zero)  blankinv=off  blankoffset=0  blankwidth=0  evsrcsel=Filtered version of DCAEVT1 (DCAEVT1FILT)  encape=off
      settings: SourceProductName=Embedded Coder Support Package for Texas Instruments C2000 Processors
  ePWM2 - ORPS2 : c2802xlib/ePWM  Commented=on  PwmType=C2000_Type4  useModule=ePWM2  ePWMxLINKTBPRD=Not Linked  periodUnits=Clock cycles  timerSource=Specify via dialog  timerPeriod_clk=1538  timerPeriod_sec=0.0001  tbshadow=Counter equals to zero  countingMode=Up-Down  phaseActiveEnable=Set counter to phase value specified via dialog  phaseDirection=Count down after sync  phaseActive=0  synchronizationEnable=off  dcaevt1Sync=off  dcbevt1Sync=off  synchronizationOption=Counter equals to zero (CTR=Zero)  perSynchronizationOption=Counter equals to zero (CTR=Zero)  clockPrescale=1  HSclockPrescale=1  enswap=off  ePWMxAStatus=on  ePWMxAactionLogic1=Do nothing  ePWMxAactionLogic2=Do nothing  ePWMxAactionLogic3=Clear  ePWMxAactionLogic4=Set  ePWMxAactionLogic5=Do nothing  ePWMxAactionLogic6=Do nothing  ePWMxACSFenable=off  ePWMxACSFvalue=Forcing disable  ePWMxASFreload=Zero  ePWMxBStatus=on  ePWMxBactionLogic1=Do nothing  ePWMxBactionLogic2=Do nothing  ePWMxBactionLogic3=Do nothing  ePWMxBactionLogic4=Do nothing  ePWMxBactionLogic5=Set  ePWMxBactionLogic6=Clear  ePWMxBCSFenable=off  ePWMxBCSFvalue=Forcing disable  ePWMxBSFreload=Zero  ePWNxBOutWay=off  ePWMxLINKCMPA=Not Linked  CMPAUnits=Clock cycles  CMPASource=Specify via dialog  CMPAValue_per=50  CMPAValue_clk=500-25  enCMPAshadow=Counter equals to zero (CTR=Zero)  ePWMxLINKCMPB=Not Linked  CMPBUnits=Clock cycles  CMPBSource=Specify via dialog  CMPBValue_per=50  CMPBValue_clk=500+25  enCMPBshadow=Counter equals to zero (CTR=Zero)  ePWMxLINKCMPC=Not Linked  CMPCUnits=Clock cycles  CMPCSource=Specify via dialog  CMPCValue_per=50  CMPCValue_clk=32000  enCMPCshadow=Counter equals to zero (CTR=Zero)  ePWMxLINKCMPD=Not Linked  CMPDUnits=Clock cycles  CMPDSource=Specify via dialog  CMPDValue_per=50  CMPDValue_clk=32000  enCMPDshadow=Counter equals to zero (CTR=Zero)  enableDBePWMxA=off  enableDBePWMxB=off  enhalfcycle=off  DBpolarity=Active high (AH)  DBedgeDelay=Positive  DBSource_ePWMxA=ePWMxA  DBSource_ePWMxB=ePWMxA  DBPeriodUnits=Clock cycles  DBperiodSource=Specify via dialog  REDperiod=0  FEDperiod=0  REDperiod_sec=0  FEDperiod_sec=0  LoadModeDBRED=Immediate without using shadow  LoadModeDBFED=Immediate without using shadow  adcstartModuleA=off  adcrequestEventA=First event  adcstartEventA=Digital Compare Module A Event 1 start of conversion (DCAEVT1.soc)  adcstartEventA_type2=Counter equals to zero (CTR=Zero)  adcstartModuleB=off  adcrequestEventB=First event  adcstartEventB=Counter equals to zero (CTR=Zero)  adcstartEventB_type2=Counter equals to zero (CTR=Zero)  intEn=off  intPrd=First event  intSel=Counter equals to zero (CTR=Zero)  intSel_type2=Counter equals to zero (CTR=Zero)  hrpe=off  enHRPWM=off  HRPWM_LoadMode=Counter equals to period (CTR=PRD)  HRPWM_CTLMode=Duty or Period control mode  HRPWM_EDGMode=Both edge  hrpeb=off  enHRPWMB=off  HRPWM_LoadModeB=Counter equals to zero (CTR=ZERO)  HRPWM_CTLModeB=Duty or Period control mode  HRPWM_EDGModeB=Both edge  enHRDBRED=off  enHRDBFED=off  enSFO=on  enautoconv=on  chopperEnable=off  chopperFrequency=1  chopperFirstwidth=1  chopperDuty=12.5%  tripZonesource=Specify via dialog  tzselOSHT1=off  tzselOSHT2=off  tzselOSHT3=off  tzselOSHDCAEV1=off  tzselOSHDCBEV1=off  tzselCBC1=off  tzselCBC2=off  tzselCBC3=off  tzselCBCDCAEV2=off  tzselCBCDCBEV2=off  tzselOSHT4=off  tzselOSHT5=off  tzselOSHT6=off  tzselCBC4=off  tzselCBC5=off  tzselCBC6=off  enTzOstIntr=off  enTzCbcIntr=off  enTzDCAEVT1Intr=off  enTzDCAEVT2Intr=off  enTzDCBEVT1Intr=off  enTzDCBEVT2Intr=off  ePWMxAforced=No action  ePWMxBforced=No action  DCAEVT1forced=No action  DCBEVT1forced=No action  DCAEVT2forced=No action  DCBEVT2forced=No action  dcah=Trip Zone 1 input (TZ1)  dcal=Trip Zone 2 input (TZ2)  dcbh=Trip Zone 1 input (TZ1)  dcbl=Trip Zone 2 input (TZ2)  dcah_type2=GPTRIP1SEL/(TZ1)  dcal_type2=GPTRIP2SEL/(TZ2)  dcbh_type2=GPTRIP1SEL/(TZ1)  dcbl_type2=GPTRIP2SEL/(TZ2)  gendcaevt1=Event disabled  gendcaevt2=Event disabled  gendcbevt1=Event disabled  gendcbevt2=Event disabled  dcaevt1src=DCAEVT1 with sync  dcaevt2src=DCAEVT2 with sync  dcbevt1src=DCBEVT1 with sync  dcbevt2src=DCBEVT2 with sync  pulsesel=Counter equals to zero (CTR=Zero)  blankinv=off  blankoffset=0  blankwidth=0  evsrcsel=Filtered version of DCAEVT1 (DCAEVT1FILT)  encape=off
      settings: SourceProductName=Embedded Coder Support Package for Texas Instruments C2000 Processors
  ePWM2 - ORPS3 : c2802xlib/ePWM  Commented=on  PwmType=C2000_Type4  useModule=ePWM2  ePWMxLINKTBPRD=Not Linked  periodUnits=Clock cycles  timerSource=Specify via dialog  timerPeriod_clk=1538  timerPeriod_sec=0.0001  tbshadow=Counter equals to zero  countingMode=Up-Down  phaseActiveEnable=Set counter to phase value specified via dialog  phaseDirection=Count down after sync  phaseActive=0  synchronizationEnable=off  dcaevt1Sync=off  dcbevt1Sync=off  synchronizationOption=Counter equals to zero (CTR=Zero)  perSynchronizationOption=Counter equals to period (CTR=PRD)  clockPrescale=1  HSclockPrescale=1  enswap=off  ePWMxAStatus=on  ePWMxAactionLogic1=Do nothing  ePWMxAactionLogic2=Do nothing  ePWMxAactionLogic3=Clear  ePWMxAactionLogic4=Set  ePWMxAactionLogic5=Do nothing  ePWMxAactionLogic6=Do nothing  ePWMxACSFenable=off  ePWMxACSFvalue=Forcing disable  ePWMxASFreload=Period  ePWMxBStatus=on  ePWMxBactionLogic1=Do nothing  ePWMxBactionLogic2=Do nothing  ePWMxBactionLogic3=Do nothing  ePWMxBactionLogic4=Do nothing  ePWMxBactionLogic5=Set  ePWMxBactionLogic6=Clear  ePWMxBCSFenable=off  ePWMxBCSFvalue=Forcing disable  ePWMxBSFreload=Period  ePWNxBOutWay=off  ePWMxLINKCMPA=Not Linked  CMPAUnits=Clock cycles  CMPASource=Specify via dialog  CMPAValue_per=50  CMPAValue_clk=769-25  enCMPAshadow=Counter equals to period (CTR=PRD)  ePWMxLINKCMPB=Not Linked  CMPBUnits=Clock cycles  CMPBSource=Specify via dialog  CMPBValue_per=50  CMPBValue_clk=769+25  enCMPBshadow=Counter equals to period (CTR=PRD)  ePWMxLINKCMPC=Not Linked  CMPCUnits=Clock cycles  CMPCSource=Specify via dialog  CMPCValue_per=50  CMPCValue_clk=500  enCMPCshadow=Counter equals to zero (CTR=Zero)  ePWMxLINKCMPD=Not Linked  CMPDUnits=Clock cycles  CMPDSource=Specify via dialog  CMPDValue_per=50  CMPDValue_clk=500  enCMPDshadow=Counter equals to zero (CTR=Zero)  enableDBePWMxA=off  enableDBePWMxB=off  enhalfcycle=off  DBpolarity=Active high (AH)  DBedgeDelay=Positive  DBSource_ePWMxA=ePWMxA  DBSource_ePWMxB=ePWMxA  DBPeriodUnits=Clock cycles  DBperiodSource=Specify via dialog  REDperiod=0  FEDperiod=0  REDperiod_sec=0  FEDperiod_sec=0  LoadModeDBRED=Immediate without using shadow  LoadModeDBFED=Immediate without using shadow  adcstartModuleA=off  adcrequestEventA=First event  adcstartEventA=Digital Compare Module A Event 1 start of conversion (DCAEVT1.soc)  adcstartEventA_type2=Counter equals to zero (CTR=Zero)  adcstartModuleB=off  adcrequestEventB=First event  adcstartEventB=Counter equals to zero (CTR=Zero)  adcstartEventB_type2=Counter equals to zero (CTR=Zero)  intEn=off  intPrd=First event  intSel=Counter equals to zero (CTR=Zero)  intSel_type2=Counter equals to zero (CTR=Zero)  hrpe=off  enHRPWM=off  HRPWM_LoadMode=Counter equals to period (CTR=PRD)  HRPWM_CTLMode=Duty or Period control mode  HRPWM_EDGMode=Both edge  hrpeb=off  enHRPWMB=off  HRPWM_LoadModeB=Counter equals to zero (CTR=ZERO)  HRPWM_CTLModeB=Duty or Period control mode  HRPWM_EDGModeB=Both edge  enHRDBRED=off  enHRDBFED=off  enSFO=on  enautoconv=on  chopperEnable=off  chopperFrequency=1  chopperFirstwidth=1  chopperDuty=12.5%  tripZonesource=Specify via dialog  tzselOSHT1=off  tzselOSHT2=off  tzselOSHT3=off  tzselOSHDCAEV1=off  tzselOSHDCBEV1=off  tzselCBC1=off  tzselCBC2=off  tzselCBC3=off  tzselCBCDCAEV2=off  tzselCBCDCBEV2=off  tzselOSHT4=off  tzselOSHT5=off  tzselOSHT6=off  tzselCBC4=off  tzselCBC5=off  tzselCBC6=off  enTzOstIntr=off  enTzCbcIntr=off  enTzDCAEVT1Intr=off  enTzDCAEVT2Intr=off  enTzDCBEVT1Intr=off  enTzDCBEVT2Intr=off  ePWMxAforced=No action  ePWMxBforced=No action  DCAEVT1forced=No action  DCBEVT1forced=No action  DCAEVT2forced=No action  DCBEVT2forced=No action  dcah=Trip Zone 1 input (TZ1)  dcal=Trip Zone 2 input (TZ2)  dcbh=Trip Zone 1 input (TZ1)  dcbl=Trip Zone 2 input (TZ2)  dcah_type2=GPTRIP1SEL/(TZ1)  dcal_type2=GPTRIP2SEL/(TZ2)  dcbh_type2=GPTRIP1SEL/(TZ1)  dcbl_type2=GPTRIP2SEL/(TZ2)  gendcaevt1=Event disabled  gendcaevt2=Event disabled  gendcbevt1=Event disabled  gendcbevt2=Event disabled  dcaevt1src=DCAEVT1 with sync  dcaevt2src=DCAEVT2 with sync  dcbevt1src=DCBEVT1 with sync  dcbevt2src=DCBEVT2 with sync  pulsesel=Counter equals to zero (CTR=Zero)  blankinv=off  blankoffset=0  blankwidth=0  evsrcsel=Filtered version of DCAEVT1 (DCAEVT1FILT)  encape=off
      settings: SourceProductName=Embedded Coder Support Package for Texas Instruments C2000 Processors
  ePWM2 - ORPS4 : c2802xlib/ePWM  PwmType=C2000_Type4  useModule=ePWM6  ePWMxLINKTBPRD=Not Linked  periodUnits=Clock cycles  timerSource=Specify via dialog  timerPeriod_clk=1538  timerPeriod_sec=0.0001  tbshadow=Counter equals to zero  countingMode=Up-Down  phaseActiveEnable=Set counter to phase value specified via dialog  phaseDirection=Count down after sync  phaseActive=0  synchronizationEnable=off  dcaevt1Sync=off  dcbevt1Sync=off  synchronizationOption=Counter equals to zero (CTR=Zero)  perSynchronizationOption=Counter equals to period (CTR=PRD)  clockPrescale=1  HSclockPrescale=1  enswap=off  ePWMxAStatus=on  ePWMxAactionLogic1=Do nothing  ePWMxAactionLogic2=Do nothing  ePWMxAactionLogic3=Clear  ePWMxAactionLogic4=Set  ePWMxAactionLogic5=Do nothing  ePWMxAactionLogic6=Do nothing  ePWMxACSFenable=off  ePWMxACSFvalue=Forcing disable  ePWMxASFreload=Period  ePWMxBStatus=on  ePWMxBactionLogic1=Do nothing  ePWMxBactionLogic2=Do nothing  ePWMxBactionLogic3=Do nothing  ePWMxBactionLogic4=Do nothing  ePWMxBactionLogic5=Set  ePWMxBactionLogic6=Clear  ePWMxBCSFenable=off  ePWMxBCSFvalue=Forcing disable  ePWMxBSFreload=Period  ePWNxBOutWay=off  ePWMxLINKCMPA=Not Linked  CMPAUnits=Clock cycles  CMPASource=Specify via dialog  CMPAValue_per=50  CMPAValue_clk=769-25  enCMPAshadow=Counter equals to period (CTR=PRD)  ePWMxLINKCMPB=Not Linked  CMPBUnits=Clock cycles  CMPBSource=Specify via dialog  CMPBValue_per=50  CMPBValue_clk=769+25  enCMPBshadow=Counter equals to period (CTR=PRD)  ePWMxLINKCMPC=Not Linked  CMPCUnits=Clock cycles  CMPCSource=Specify via dialog  CMPCValue_per=50  CMPCValue_clk=500  enCMPCshadow=Counter equals to zero (CTR=Zero)  ePWMxLINKCMPD=Not Linked  CMPDUnits=Clock cycles  CMPDSource=Specify via dialog  CMPDValue_per=50  CMPDValue_clk=500  enCMPDshadow=Counter equals to zero (CTR=Zero)  enableDBePWMxA=off  enableDBePWMxB=off  enhalfcycle=off  DBpolarity=Active high (AH)  DBedgeDelay=Positive  DBSource_ePWMxA=ePWMxA  DBSource_ePWMxB=ePWMxA  DBPeriodUnits=Clock cycles  DBperiodSource=Specify via dialog  REDperiod=0  FEDperiod=0  REDperiod_sec=0  FEDperiod_sec=0  LoadModeDBRED=Immediate without using shadow  LoadModeDBFED=Immediate without using shadow  adcstartModuleA=off  adcrequestEventA=First event  adcstartEventA=Digital Compare Module A Event 1 start of conversion (DCAEVT1.soc)  adcstartEventA_type2=Counter equals to zero (CTR=Zero)  adcstartModuleB=off  adcrequestEventB=First event  adcstartEventB=Counter equals to zero (CTR=Zero)  adcstartEventB_type2=Counter equals to zero (CTR=Zero)  intEn=off  intPrd=First event  intSel=Counter equals to zero (CTR=Zero)  intSel_type2=Counter equals to zero (CTR=Zero)  hrpe=off  enHRPWM=off  HRPWM_LoadMode=Counter equals to period (CTR=PRD)  HRPWM_CTLMode=Duty or Period control mode  HRPWM_EDGMode=Both edge  hrpeb=off  enHRPWMB=off  HRPWM_LoadModeB=Counter equals to zero (CTR=ZERO)  HRPWM_CTLModeB=Duty or Period control mode  HRPWM_EDGModeB=Both edge  enHRDBRED=off  enHRDBFED=off  enSFO=on  enautoconv=on  chopperEnable=off  chopperFrequency=1  chopperFirstwidth=1  chopperDuty=12.5%  tripZonesource=Specify via dialog  tzselOSHT1=off  tzselOSHT2=off  tzselOSHT3=off  tzselOSHDCAEV1=off  tzselOSHDCBEV1=off  tzselCBC1=off  tzselCBC2=off  tzselCBC3=off  tzselCBCDCAEV2=off  tzselCBCDCBEV2=off  tzselOSHT4=off  tzselOSHT5=off  tzselOSHT6=off  tzselCBC4=off  tzselCBC5=off  tzselCBC6=off  enTzOstIntr=off  enTzCbcIntr=off  enTzDCAEVT1Intr=off  enTzDCAEVT2Intr=off  enTzDCBEVT1Intr=off  enTzDCBEVT2Intr=off  ePWMxAforced=No action  ePWMxBforced=No action  DCAEVT1forced=No action  DCBEVT1forced=No action  DCAEVT2forced=No action  DCBEVT2forced=No action  dcah=Trip Zone 1 input (TZ1)  dcal=Trip Zone 2 input (TZ2)  dcbh=Trip Zone 1 input (TZ1)  dcbl=Trip Zone 2 input (TZ2)  dcah_type2=GPTRIP1SEL/(TZ1)  dcal_type2=GPTRIP2SEL/(TZ2)  dcbh_type2=GPTRIP1SEL/(TZ1)  dcbl_type2=GPTRIP2SEL/(TZ2)  gendcaevt1=Event disabled  gendcaevt2=Event disabled  gendcbevt1=Event disabled  gendcbevt2=Event disabled  dcaevt1src=DCAEVT1 with sync  dcaevt2src=DCAEVT2 with sync  dcbevt1src=DCBEVT1 with sync  dcbevt2src=DCBEVT2 with sync  pulsesel=Counter equals to zero (CTR=Zero)  blankinv=off  blankoffset=0  blankwidth=0  evsrcsel=Filtered version of DCAEVT1 (DCAEVT1FILT)  encape=off
      settings: SourceProductName=Embedded Coder Support Package for Texas Instruments C2000 Processors
